simulink model "Robust_PID"  (R2017b)
settings: Solver=ode5  StartTime=0.0  StopTime=10.0  FixedStep=0.0001  RelTol=1e-3
values from neighbouring files (symbols this model uses):
  aa = 10    [Robust_PSOPID.m]    (also in Robust_PSOPID_PI.m)
  bb = 7    [Robust_PSOPID.m]    (also in Robust_PSOPID_PI.m)
  cc = 8    [Robust_PSOPID.m]    (also in Robust_PSOPID_PI.m)
  Kd = swarm(i, 3, 3)    [PSOEXPID1.m]    (also in PSO_fitfun_EXPID1.m = particle(3); Robust_PSOPID.m = swarm(gbest_pos, 3, 3); Robust_PSOPID_PI.m = PID(3))
  Ki = swarm(i, 3, 2)    [PSOEXPID1.m]    (also in PSO_fitfun_EXPID1.m = particle(2); Robust_PSOPID.m = swarm(gbest_pos, 3, 2); Robust_PSOPID_PI.m = PID(2))
  Kp = swarm(i, 3, 1)    [PSOEXPID1.m]    (also in PSO_fitfun_EXPID1.m = particle(1); Robust_PSOPID.m = swarm(gbest_pos, 3, 1); Robust_PSOPID_PI.m = PID(1))
settings Model: Creator=Yenchun  LastModifiedBy=liyenjun
settings CodeAppCC: StateflowObjectComments=on

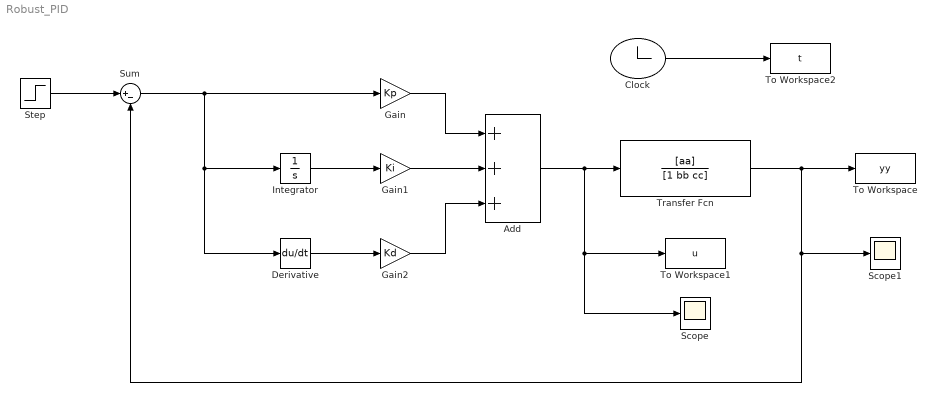
== system Robust_PID ==
  Add : Sum  Inputs=+++
  Clock : Clock
  Derivative : Derivative
  Gain : Gain  Gain=Kp
  Gain1 : Gain  Gain=Ki
  Gain2 : Gain  Gain=Kd
  Integrator : Integrator
  Scope : Scope
  Scope1 : Scope
  Step : Step  Before=1  SampleTime=0
  Sum : Sum  Inputs=|+-
  To Workspace : ToWorkspace  VariableName=yy  SampleTime=-1
      settings: Save2DSignal=2-D array (concatenate along first dimension)
  To Workspace1 : ToWorkspace  VariableName=u  SampleTime=-1
      settings: Save2DSignal=2-D array (concatenate along first dimension)
  To Workspace2 : ToWorkspace  VariableName=t  SampleTime=-1
      settings: Save2DSignal=2-D array (concatenate along first dimension)
  Transfer Fcn : TransferFcn  Numerator=[aa]  Denominator=[1 bb cc]
  wires:
  Step/1 -> Sum/1
  Integrator/1 -> Gain1/1
  Derivative/1 -> Gain2/1
  Sum/1 -> Derivative/1, Integrator/1, Gain/1
  Gain/1 -> Add/1
  Gain1/1 -> Add/2
  Gain2/1 -> Add/3
  Add/1 -> Scope/1, To Workspace1/1, Transfer Fcn/1
  Transfer Fcn/1 -> To Workspace/1, Scope1/1, Sum/2
  Clock/1 -> To Workspace2/1
